simulink model "ep4_1"  (R2018a)
settings: Solver=VariableStepAuto  StartTime=0.0  StopTime=50  MaxStep=0.01  RelTol=1e-3
settings Model: Creator=zheny  LastModifiedBy=zheny

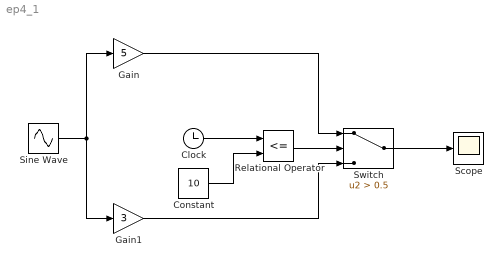
== system ep4_1 ==
  Clock : Clock
  Constant : Constant  Value=10
  Gain : Gain  Gain=5
  Gain1 : Gain  Gain=3
  Relational Operator : RelationalOperator  Operator=<=  OutDataTypeStr=boolean  RndMeth=Simplest
  Scope : Scope
  Sine Wave : Sin  SampleTime=0
  Switch : Switch  Criteria=u2 > Threshold  Threshold=0.5
  wires:
  Relational Operator/1 -> Switch/2
  Sine Wave/1 -> Gain1/1, Gain/1
  Clock/1 -> Relational Operator/1
  Constant/1 -> Relational Operator/2
  Gain/1 -> Switch/1
  Gain1/1 -> Switch/3
  Switch/1 -> Scope/1
